simulink model "speedChange_fsm"  (R2022a)
settings: Solver=FixedStepDiscrete  StartTime=0.0  StopTime=10.0  FixedStep=0.1  RelTol=1e-3  EnableMultiTasking=on
settings Model: Creator=steve  LastModifiedBy=Nate
settings SolverCC: AlgebraicLoopSolver=TrustRegion  AutoInsertRateTranBlk=on
settings DataIOCC: LimitDataPoints=on
settings OptimizationCC: LifeSpan=inf
settings DebuggingCC: UnconnectedInputMsg=warning  UnconnectedOutputMsg=warning  UnconnectedLineMsg=warning  AllowSymbolicDim=off  SFUnexpectedBacktrackingDiag=warning  SFNoUnconditionalDefaultTransitionDiag=warning  SFExecutionAtInitializationDiag=none  ArithmeticOperatorsInVariantConditions=warning
settings SFSimCC: SimUseLocalCustomCode=off  CustomCodeUndefinedFunction=UseInterfaceOnly
settings RTWCC: RTWUseLocalCustomCode=off  DLArmComputeVersion=19.05
settings CodeAppCC: StateflowObjectComments=on
settings GRTTargetCC: TargetLangStandard=C89/C90 (ANSI)
settings ConfigComp: CovMetricSettings=dw  CovSaveCumulativeToWorkspaceVar=on  CovSaveSingleToWorkspaceVar=on  CovExternalEMLEnable=off  CovSFcnEnable=off

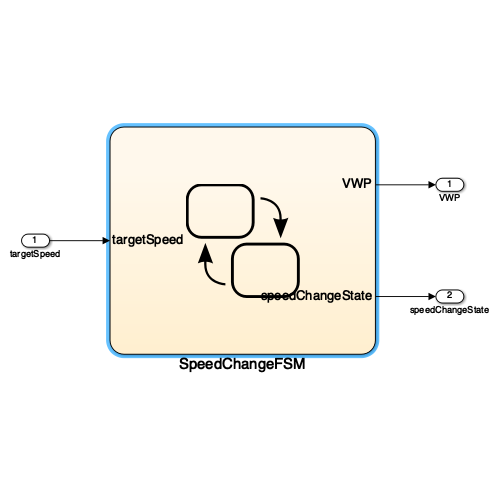
[thumbnail: Simulink's stored preview of the top-level diagram]
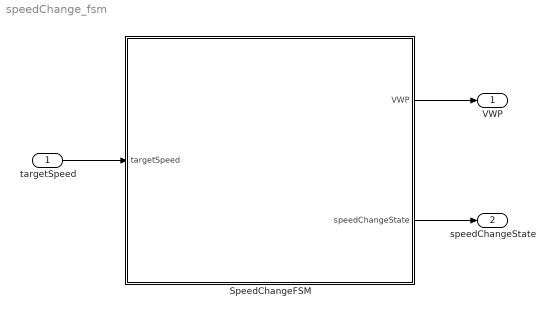
== system speedChange_fsm ==
  targetSpeed : Inport
  SpeedChangeFSM : Stateflow chart  TreatAsAtomicUnit=on
  VWP : Outport
  speedChangeState : Outport  Port=2
  wires:
  targetSpeed/1 -> SpeedChangeFSM/1(targetSpeed)
  SpeedChangeFSM/2(speedChangeState) -> speedChangeState/1
  SpeedChangeFSM/1(VWP) -> VWP/1

== stateflow chart speedChange_fsm/SpeedChangeFSM ==
  state wait_for_speedChange_enable
    en:  speedChangeState = 0;
  state wait_for_stop_duration
    en:  speedChangeState = 1;
  (default) -> wait_for_speedChange_enable
  wait_for_speedChange_enable -> wait_for_speedChange_enable [order 2]
  wait_for_stop_duration -> wait_for_speedChange_enable [order 1] : [SpeedChangeEnable == false || ...
      |   abs(vCar - targetSpeed) < 0.1]
      | {SubMachineRunning = false && ...
      | SpeedChangeEnable == false}
  wait_for_speedChange_enable -> wait_for_stop_duration [order 1] : [SpeedChangeEnable == true]
      | {VWP = updateVehicleSpeed(VWP, targetSpeed)}
  wait_for_stop_duration -> wait_for_stop_duration [order 2]
  data: VWP output; SpeedChangeEnable data_store_memory; targetSpeed input; SubMachineRunning data_store_memory; speedChangeState output; vCar local
